simulink model "TCMSSystem"  (R2019b)
settings: configuration reference "ConfigSet_TCMSSystem_Reference" (kept outside this file)
model workspace (MAT data in the model file):
  Prm_TCMSSystem : Simulink.Parameter (value not decoded)
  SampleTime = 0.05
symbols that are objects in the model workspace (value not decoded): Prm_TCMSSystem
undefined symbols (not defined in the file): ADDIntervention, AK1Status, AK2Status, AKContactorStatus, AllDoorsClosed, AllLeftDoorsClosed, AllRightDoorsClosed, APS1Fault, APS1Isolated, APS1OutputVoltage, APS1Status, APS2Fault, APS2Isolated, APS2OutputVoltage, APS2Status, APSKAKContactor, ASCOEnd1, ASCOEnd2, ATBMode, ATCBypassMode, ATCStatusNotOK, ATOMode, ATPLowSpeedCutoutStatus, ATPMode, AuxCompressor, BatteryCurrent, BatteryIsolationContactor, BatteryTemperature, BatteryVoltage, BCG1Fault, BCG1Isolated, BCG1IsolationFailed, BCG1OutputCurrent, BCG1Status, BCG2Fault, BCG2Isolated, BCG2OutputCurrent, BCG2Status, BCGOutputVoltage, BECU1AxleLockedWheelSet1, BECU2AxleLockedWheelSet2, BECUFaulty, BECUMajorFault, BECUMinorFault, BECUStatus, BIC1Inside, BIC1Outside, BIC2Inside, BIC2Outside, Bogie, Bogie1WSPStatus, Bogie2WSPStatus, BogieFaulty, BogieIsolationStatus, BogieSupportedMass, BrakeCylinderPressureGauge, BrakeLoopCBTripped, BrakeLoopOpenTL, BrakeTrainLineStatus, BrakingDemand ... (+215)
libraries: TimersLib x257, simulink x137, LatchesLib x42, VectorOperationsLib x15, TestBenchLib x12, MathOperationsLib x2, FiltersLib x1
(part 10 of 16)

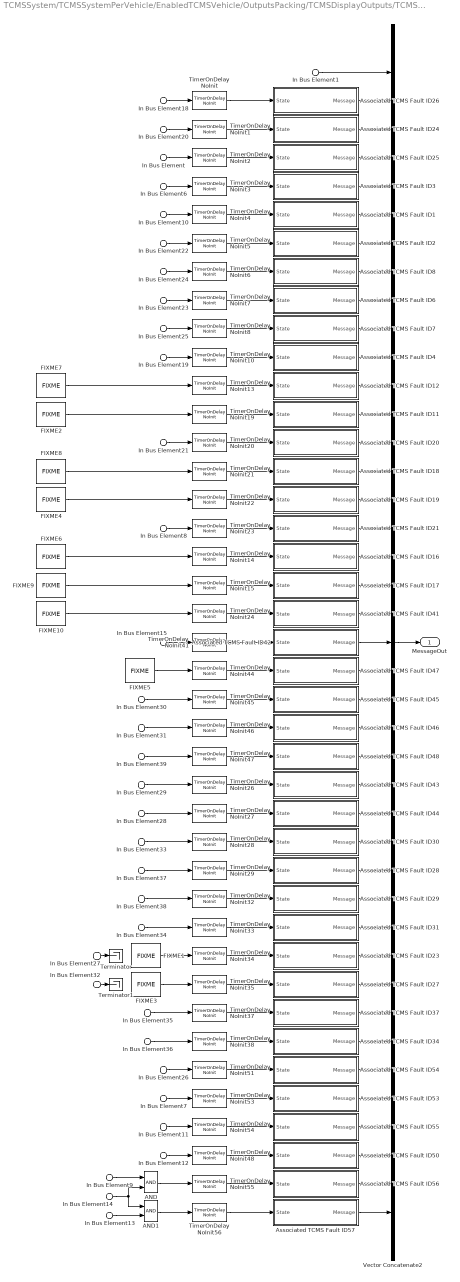
== system TCMSSystem/TCMSSystemPerVehicle/EnabledTCMSVehicle/OutputsPacking/TCMSDisplayOutputs/TCMSMessageEvents/New46EventsMessage ==
  In Bus Element1 : Inport  PortName=MessageIn
  In Bus Element15 : Inport  Port=2  PortName=BusIn  Element=PantographSystem.PantographIsolated
  In Bus Element : Inport  Port=2  PortName=BusIn  Element=ElectricalSystem.BrakeLoopCBTripped
  In Bus Element12 : Inport  Port=2  PortName=BusIn  Element=ElectricalSystem.VCBIsolated
  In Bus Element19 : Inport  Port=2  PortName=BusIn  Element=ElectricalSystem.APS2Isolated
  In Bus Element14 : Inport  Port=2  PortName=BusIn  Element=ElectricalSystem.CabActive
  In Bus Element6 : Inport  Port=2  PortName=BusIn  Element=PneumaticsSystem.Bogie1ParkingBrakeIsolated
  In Bus Element10 : Inport  Port=2  PortName=BusIn  Element=PneumaticsSystem.Bogie2ParkingBrakeIsolated
  In Bus Element8 : Inport  Port=3  PortName=ElectricalControl  Element=BLCOSwitchStatus
  In Bus Element9 : Inport  Port=3  PortName=ElectricalControl  Element=TooManyBogiesIsolated
  In Bus Element13 : Inport  Port=3  PortName=ElectricalControl  Element=TooManyEPICCutout
  In Bus Element26 : Inport  Port=3  PortName=ElectricalControl  Element=WFLIsolated
  In Bus Element27 : Inport  Port=3  PortName=ElectricalControl  Element=HVAC1FireDetectorDisableVDUReq
  In Bus Element28 : Inport  Port=3  PortName=ElectricalControl  Element=EDBHeatAlarmDisableVDUReq
  In Bus Element29 : Inport  Port=3  PortName=ElectricalControl  Element=CABSmokeDetectorDisableVDUReq
  In Bus Element30 : Inport  Port=3  PortName=ElectricalControl  Element=SHDEndCubicleRearRight1DisableVDUReq
  In Bus Element31 : Inport  Port=3  PortName=ElectricalControl  Element=SHDEndCubicleRearRight2DisableVDUReq
  In Bus Element32 : Inport  Port=3  PortName=ElectricalControl  Element=SHDEndCubicleRearLeft1DisableVDUReq
  In Bus Element33 : Inport  Port=3  PortName=ElectricalControl  Element=SHDEndCubicleRearLeft2DisableVDUReq
  In Bus Element34 : Inport  Port=3  PortName=ElectricalControl  Element=LHDDriverDeskDisableVDUReq
  In Bus Element35 : Inport  Port=3  PortName=ElectricalControl  Element=LHDCIDisableVDUReq
  In Bus Element36 : Inport  Port=3  PortName=ElectricalControl  Element=LHDLTJBDisableVDUReq
  In Bus Element37 : Inport  Port=3  PortName=ElectricalControl  Element=SaloonR1FireDetectorDisableVDUReq
  In Bus Element38 : Inport  Port=3  PortName=ElectricalControl  Element=SaloonR2FireDetectorDisableVDUReq
  In Bus Element39 : Inport  Port=3  PortName=ElectricalControl  Element=AuxiliaryDeskFireDetectorDisableVDUReq
  In Bus Element7 : Inport  Port=3  PortName=ElectricalControl  Element=RemoteMagnetValve1
  In Bus Element11 : Inport  Port=3  PortName=ElectricalControl  Element=RemoteMagnetValve2
  In Bus Element18 : Inport  Port=4  PortName=PneumaticsControl  Element=ASCOEnd1
  In Bus Element20 : Inport  Port=4  PortName=PneumaticsControl  Element=ASCOEnd2
  In Bus Element21 : Inport  Port=4  PortName=PneumaticsControl  Element=HornManuallyIsolated
  In Bus Element22 : Inport  Port=4  PortName=PneumaticsControl  Element=BIC1Inside
  In Bus Element23 : Inport  Port=4  PortName=PneumaticsControl  Element=BIC1Outside
  In Bus Element24 : Inport  Port=4  PortName=PneumaticsControl  Element=BIC2Inside
  In Bus Element25 : Inport  Port=4  PortName=PneumaticsControl  Element=BIC2Outside
  AND : Logic  AllPortsSameDT=off  OutDataTypeStr=boolean
  AND1 : Logic  AllPortsSameDT=off  OutDataTypeStr=boolean
  Associated TCMS Fault ID1 : Subsystem  mask{MessageID=91031}
      mask Display:
      | port_label('output', 1, ['ID = ' num2str(MessageID)])
      | port_label('input', 1, 'Status')
  Associated TCMS Fault ID11 : Subsystem  mask{MessageID=3006}
      mask Display:
      | port_label('output', 1, ['ID = ' num2str(MessageID)])
      | port_label('input', 1, 'Status')
  Associated TCMS Fault ID12 : Subsystem  mask{MessageID=241003}
      mask Display:
      | port_label('output', 1, ['ID = ' num2str(MessageID)])
      | port_label('input', 1, 'Status')
  Associated TCMS Fault ID16 : Subsystem  mask{MessageID=91044}
      mask Display:
      | port_label('output', 1, ['ID = ' num2str(MessageID)])
      | port_label('input', 1, 'Status')
  Associated TCMS Fault ID17 : Subsystem  mask{MessageID=12103}
      mask Display:
      | port_label('output', 1, ['ID = ' num2str(MessageID)])
      | port_label('input', 1, 'Status')
  Associated TCMS Fault ID18 : Subsystem  mask{MessageID=1010}
      mask Display:
      | port_label('output', 1, ['ID = ' num2str(MessageID)])
      | port_label('input', 1, 'Status')
  Associated TCMS Fault ID19 : Subsystem  mask{MessageID=1008}
      mask Display:
      | port_label('output', 1, ['ID = ' num2str(MessageID)])
      | port_label('input', 1, 'Status')
  Associated TCMS Fault ID2 : Subsystem  mask{MessageID=91026}
      mask Display:
      | port_label('output', 1, ['ID = ' num2str(MessageID)])
      | port_label('input', 1, 'Status')
  Associated TCMS Fault ID20 : Subsystem  mask{MessageID=1009}
      mask Display:
      | port_label('output', 1, ['ID = ' num2str(MessageID)])
      | port_label('input', 1, 'Status')
  Associated TCMS Fault ID21 : Subsystem  mask{MessageID=91022}
      mask Display:
      | port_label('output', 1, ['ID = ' num2str(MessageID)])
      | port_label('input', 1, 'Status')
  Associated TCMS Fault ID23 : Subsystem  mask{MessageID=151078}
      mask Display:
      | port_label('output', 1, ['ID = ' num2str(MessageID)])
      | port_label('input', 1, 'Status')
  Associated TCMS Fault ID24 : Subsystem  mask{MessageID=91033}
      mask Display:
      | port_label('output', 1, ['ID = ' num2str(MessageID)])
      | port_label('input', 1, 'Status')
  Associated TCMS Fault ID25 : Subsystem  mask{MessageID=93055}
      mask Display:
      | port_label('output', 1, ['ID = ' num2str(MessageID)])
      | port_label('input', 1, 'Status')
  Associated TCMS Fault ID26 : Subsystem  mask{MessageID=91032}
      mask Display:
      | port_label('output', 1, ['ID = ' num2str(MessageID)])
      | port_label('input', 1, 'Status')
  Associated TCMS Fault ID27 : Subsystem  mask{MessageID=151079}
      mask Display:
      | port_label('output', 1, ['ID = ' num2str(MessageID)])
      | port_label('input', 1, 'Status')
  Associated TCMS Fault ID28 : Subsystem  mask{MessageID=151067}
      mask Display:
      | port_label('output', 1, ['ID = ' num2str(MessageID)])
      | port_label('input', 1, 'Status')
  Associated TCMS Fault ID29 : Subsystem  mask{MessageID=151068}
      mask Display:
      | port_label('output', 1, ['ID = ' num2str(MessageID)])
      | port_label('input', 1, 'Status')
  Associated TCMS Fault ID3 : Subsystem  mask{MessageID=91030}
      mask Display:
      | port_label('output', 1, ['ID = ' num2str(MessageID)])
      | port_label('input', 1, 'Status')
  Associated TCMS Fault ID30 : Subsystem  mask{MessageID=151066}
      mask Display:
      | port_label('output', 1, ['ID = ' num2str(MessageID)])
      | port_label('input', 1, 'Status')
  Associated TCMS Fault ID31 : Subsystem  mask{MessageID=151077}
      mask Display:
      | port_label('output', 1, ['ID = ' num2str(MessageID)])
      | port_label('input', 1, 'Status')
  Associated TCMS Fault ID34 : Subsystem  mask{MessageID=151090}
      mask Display:
      | port_label('output', 1, ['ID = ' num2str(MessageID)])
      | port_label('input', 1, 'Status')
  Associated TCMS Fault ID37 : Subsystem  mask{MessageID=151089}
      mask Display:
      | port_label('output', 1, ['ID = ' num2str(MessageID)])
      | port_label('input', 1, 'Status')
  Associated TCMS Fault ID4 : Subsystem  mask{MessageID=232005}
      mask Display:
      | port_label('output', 1, ['ID = ' num2str(MessageID)])
      | port_label('input', 1, 'Status')
  Associated TCMS Fault ID41 : Subsystem  mask{MessageID=12104}
      mask Display:
      | port_label('output', 1, ['ID = ' num2str(MessageID)])
      | port_label('input', 1, 'Status')
  Associated TCMS Fault ID42 : Subsystem  mask{MessageID=12007}
      mask Display:
      | port_label('output', 1, ['ID = ' num2str(MessageID)])
      | port_label('input', 1, 'Status')
  Associated TCMS Fault ID43 : Subsystem  mask{MessageID=151064}
      mask Display:
      | port_label('output', 1, ['ID = ' num2str(MessageID)])
      | port_label('input', 1, 'Status')
  Associated TCMS Fault ID44 : Subsystem  mask{MessageID=151065}
      mask Display:
      | port_label('output', 1, ['ID = ' num2str(MessageID)])
      | port_label('input', 1, 'Status')
  Associated TCMS Fault ID45 : Subsystem  mask{MessageID=151061}
      mask Display:
      | port_label('output', 1, ['ID = ' num2str(MessageID)])
      | port_label('input', 1, 'Status')
  Associated TCMS Fault ID46 : Subsystem  mask{MessageID=151062}
      mask Display:
      | port_label('output', 1, ['ID = ' num2str(MessageID)])
      | port_label('input', 1, 'Status')
  Associated TCMS Fault ID47 : Subsystem  mask{MessageID=30035}
      mask Display:
      | port_label('output', 1, ['ID = ' num2str(MessageID)])
      | port_label('input', 1, 'Status')
  Associated TCMS Fault ID48 : Subsystem  mask{MessageID=151063}
      mask Display:
      | port_label('output', 1, ['ID = ' num2str(MessageID)])
      | port_label('input', 1, 'Status')
  Associated TCMS Fault ID50 : Subsystem  mask{MessageID=12014}
      mask Display:
      | port_label('output', 1, ['ID = ' num2str(MessageID)])
      | port_label('input', 1, 'Status')
  Associated TCMS Fault ID53 : Subsystem  mask{MessageID=91036}
      mask Display:
      | port_label('output', 1, ['ID = ' num2str(MessageID)])
      | port_label('input', 1, 'Status')
  Associated TCMS Fault ID54 : Subsystem  mask{MessageID=261006}
      mask Display:
      | port_label('output', 1, ['ID = ' num2str(MessageID)])
      | port_label('input', 1, 'Status')
  Associated TCMS Fault ID55 : Subsystem  mask{MessageID=91037}
      mask Display:
      | port_label('output', 1, ['ID = ' num2str(MessageID)])
      | port_label('input', 1, 'Status')
  Associated TCMS Fault ID56 : Subsystem  mask{MessageID=888888}
      mask Display:
      | port_label('output', 1, ['ID = ' num2str(MessageID)])
      | port_label('input', 1, 'Status')
  Associated TCMS Fault ID57 : Subsystem  mask{MessageID=999999}
      mask Display:
      | port_label('output', 1, ['ID = ' num2str(MessageID)])
      | port_label('input', 1, 'Status')
  Associated TCMS Fault ID6 : Subsystem  mask{MessageID=91028}
      mask Display:
      | port_label('output', 1, ['ID = ' num2str(MessageID)])
      | port_label('input', 1, 'Status')
  Associated TCMS Fault ID7 : Subsystem  mask{MessageID=91029}
      mask Display:
      | port_label('output', 1, ['ID = ' num2str(MessageID)])
      | port_label('input', 1, 'Status')
  Associated TCMS Fault ID8 : Subsystem  mask{MessageID=91027}
      mask Display:
      | port_label('output', 1, ['ID = ' num2str(MessageID)])
      | port_label('input', 1, 'Status')
  FIXME{1..10} (10 alike) : TestBenchLib/FIXME
      settings: SourceProductName=Sydac Utilities
  Terminator : Terminator
  Terminator1 : Terminator
  TimerOnDelay NoInit{,1..8,10,13..15,19..24,26..29,32..35,37..38,41,44..48,51,53..56} (40 alike) : TimersLib/TimerOnDelay NoInit  UpperSaturationLimit=0.5  OutputTime=off  SampleTime=-1
      settings: SourceProductName=Sydac Utilities
  Vector Concatenate2 : Concatenate  NumInputs=41
  MessageOut : Outport
  wires:
  TimerOnDelay NoInit2/1 -> Associated TCMS Fault ID25/1(State)
  TimerOnDelay NoInit1/1 -> Associated TCMS Fault ID24/1(State)
  TimerOnDelay NoInit/1 -> Associated TCMS Fault ID26/1(State)
  In Bus Element1/1 -> Vector Concatenate2/1
  Associated TCMS Fault ID25/1(Message) -> Vector Concatenate2/4
  Associated TCMS Fault ID26/1(Message) -> Vector Concatenate2/2
  In Bus Element/1 -> TimerOnDelay NoInit2/1
  Vector Concatenate2/1 -> MessageOut/1
  Associated TCMS Fault ID24/1(Message) -> Vector Concatenate2/3
  Associated TCMS Fault ID1/1(Message) -> Vector Concatenate2/6
  Associated TCMS Fault ID3/1(Message) -> Vector Concatenate2/5
  Associated TCMS Fault ID2/1(Message) -> Vector Concatenate2/7
  TimerOnDelay NoInit3/1 -> Associated TCMS Fault ID3/1(State)
  TimerOnDelay NoInit4/1 -> Associated TCMS Fault ID1/1(State)
  TimerOnDelay NoInit5/1 -> Associated TCMS Fault ID2/1(State)
  TimerOnDelay NoInit10/1 -> Associated TCMS Fault ID4/1(State)
  In Bus Element19/1 -> TimerOnDelay NoInit10/1
  Associated TCMS Fault ID6/1(Message) -> Vector Concatenate2/9
  Associated TCMS Fault ID8/1(Message) -> Vector Concatenate2/8
  Associated TCMS Fault ID7/1(Message) -> Vector Concatenate2/10
  TimerOnDelay NoInit6/1 -> Associated TCMS Fault ID8/1(State)
  TimerOnDelay NoInit7/1 -> Associated TCMS Fault ID6/1(State)
  TimerOnDelay NoInit8/1 -> Associated TCMS Fault ID7/1(State)
  TimerOnDelay NoInit22/1 -> Associated TCMS Fault ID19/1(State)
  TimerOnDelay NoInit21/1 -> Associated TCMS Fault ID18/1(State)
  TimerOnDelay NoInit20/1 -> Associated TCMS Fault ID20/1(State)
  FIXME2/1 -> TimerOnDelay NoInit19/1
  FIXME8/1 -> TimerOnDelay NoInit21/1
  FIXME6/1 -> TimerOnDelay NoInit14/1
  FIXME9/1 -> TimerOnDelay NoInit15/1
  TimerOnDelay NoInit23/1 -> Associated TCMS Fault ID21/1(State)
  TimerOnDelay NoInit14/1 -> Associated TCMS Fault ID16/1(State)
  TimerOnDelay NoInit15/1 -> Associated TCMS Fault ID17/1(State)
  TimerOnDelay NoInit19/1 -> Associated TCMS Fault ID11/1(State)
  FIXME7/1 -> TimerOnDelay NoInit13/1
  TimerOnDelay NoInit13/1 -> Associated TCMS Fault ID12/1(State)
  TimerOnDelay NoInit32/1 -> Associated TCMS Fault ID29/1(State)
  TimerOnDelay NoInit29/1 -> Associated TCMS Fault ID28/1(State)
  TimerOnDelay NoInit28/1 -> Associated TCMS Fault ID30/1(State)
  TimerOnDelay NoInit33/1 -> Associated TCMS Fault ID31/1(State)
  TimerOnDelay NoInit34/1 -> Associated TCMS Fault ID23/1(State)
  TimerOnDelay NoInit35/1 -> Associated TCMS Fault ID27/1(State)
  FIXME5/1 -> TimerOnDelay NoInit44/1
  TimerOnDelay NoInit37/1 -> Associated TCMS Fault ID37/1(State)
  TimerOnDelay NoInit38/1 -> Associated TCMS Fault ID34/1(State)
  TimerOnDelay NoInit46/1 -> Associated TCMS Fault ID46/1(State)
  TimerOnDelay NoInit45/1 -> Associated TCMS Fault ID45/1(State)
  TimerOnDelay NoInit44/1 -> Associated TCMS Fault ID47/1(State)
  TimerOnDelay NoInit47/1 -> Associated TCMS Fault ID48/1(State)
  TimerOnDelay NoInit26/1 -> Associated TCMS Fault ID43/1(State)
  TimerOnDelay NoInit27/1 -> Associated TCMS Fault ID44/1(State)
  TimerOnDelay NoInit41/1 -> Associated TCMS Fault ID42/1(State)
  TimerOnDelay NoInit24/1 -> Associated TCMS Fault ID41/1(State)
  TimerOnDelay NoInit53/1 -> Associated TCMS Fault ID53/1(State)
  TimerOnDelay NoInit51/1 -> Associated TCMS Fault ID54/1(State)
  TimerOnDelay NoInit54/1 -> Associated TCMS Fault ID55/1(State)
  TimerOnDelay NoInit48/1 -> Associated TCMS Fault ID50/1(State)
  TimerOnDelay NoInit56/1 -> Associated TCMS Fault ID57/1(State)
  TimerOnDelay NoInit55/1 -> Associated TCMS Fault ID56/1(State)
  Associated TCMS Fault ID4/1(Message) -> Vector Concatenate2/11
  Associated TCMS Fault ID12/1(Message) -> Vector Concatenate2/12
  Associated TCMS Fault ID11/1(Message) -> Vector Concatenate2/13
  Associated TCMS Fault ID20/1(Message) -> Vector Concatenate2/14
  Associated TCMS Fault ID18/1(Message) -> Vector Concatenate2/15
  Associated TCMS Fault ID19/1(Message) -> Vector Concatenate2/16
  Associated TCMS Fault ID21/1(Message) -> Vector Concatenate2/17
  Associated TCMS Fault ID16/1(Message) -> Vector Concatenate2/18
  Associated TCMS Fault ID17/1(Message) -> Vector Concatenate2/19
  Associated TCMS Fault ID41/1(Message) -> Vector Concatenate2/20
  Associated TCMS Fault ID42/1(Message) -> Vector Concatenate2/21
  Associated TCMS Fault ID47/1(Message) -> Vector Concatenate2/22
  Associated TCMS Fault ID45/1(Message) -> Vector Concatenate2/23
  Associated TCMS Fault ID46/1(Message) -> Vector Concatenate2/24
  Associated TCMS Fault ID48/1(Message) -> Vector Concatenate2/25
  Associated TCMS Fault ID43/1(Message) -> Vector Concatenate2/26
  Associated TCMS Fault ID44/1(Message) -> Vector Concatenate2/27
  Associated TCMS Fault ID30/1(Message) -> Vector Concatenate2/28
  Associated TCMS Fault ID28/1(Message) -> Vector Concatenate2/29
  Associated TCMS Fault ID29/1(Message) -> Vector Concatenate2/30
  Associated TCMS Fault ID31/1(Message) -> Vector Concatenate2/31
  Associated TCMS Fault ID23/1(Message) -> Vector Concatenate2/32
  Associated TCMS Fault ID27/1(Message) -> Vector Concatenate2/33
  Associated TCMS Fault ID37/1(Message) -> Vector Concatenate2/34
  Associated TCMS Fault ID34/1(Message) -> Vector Concatenate2/35
  Associated TCMS Fault ID54/1(Message) -> Vector Concatenate2/36
  Associated TCMS Fault ID53/1(Message) -> Vector Concatenate2/37
  Associated TCMS Fault ID55/1(Message) -> Vector Concatenate2/38
  Associated TCMS Fault ID50/1(Message) -> Vector Concatenate2/39
  Associated TCMS Fault ID56/1(Message) -> Vector Concatenate2/40
  Associated TCMS Fault ID57/1(Message) -> Vector Concatenate2/41
  In Bus Element6/1 -> TimerOnDelay NoInit3/1
  In Bus Element10/1 -> TimerOnDelay NoInit4/1
  In Bus Element15/1 -> TimerOnDelay NoInit41/1
  In Bus Element7/1 -> TimerOnDelay NoInit53/1
  In Bus Element11/1 -> TimerOnDelay NoInit54/1
  FIXME10/1 -> TimerOnDelay NoInit24/1
  In Bus Element12/1 -> TimerOnDelay NoInit48/1
  FIXME4/1 -> TimerOnDelay NoInit22/1
  In Bus Element8/1 -> TimerOnDelay NoInit23/1
  In Bus Element9/1 -> AND/1
  In Bus Element13/1 -> AND1/2
  In Bus Element14/1 -> AND1/1, AND/2
  AND/1 -> TimerOnDelay NoInit55/1
  AND1/1 -> TimerOnDelay NoInit56/1
  In Bus Element18/1 -> TimerOnDelay NoInit/1
  In Bus Element20/1 -> TimerOnDelay NoInit1/1
  In Bus Element21/1 -> TimerOnDelay NoInit20/1
  In Bus Element22/1 -> TimerOnDelay NoInit5/1
  In Bus Element23/1 -> TimerOnDelay NoInit7/1
  In Bus Element24/1 -> TimerOnDelay NoInit6/1
  In Bus Element25/1 -> TimerOnDelay NoInit8/1
  In Bus Element26/1 -> TimerOnDelay NoInit51/1
  In Bus Element30/1 -> TimerOnDelay NoInit45/1
  In Bus Element31/1 -> TimerOnDelay NoInit46/1
  In Bus Element39/1 -> TimerOnDelay NoInit47/1
  In Bus Element29/1 -> TimerOnDelay NoInit26/1
  In Bus Element28/1 -> TimerOnDelay NoInit27/1
  In Bus Element33/1 -> TimerOnDelay NoInit28/1
  In Bus Element37/1 -> TimerOnDelay NoInit29/1
  In Bus Element38/1 -> TimerOnDelay NoInit32/1
  In Bus Element34/1 -> TimerOnDelay NoInit33/1
  In Bus Element35/1 -> TimerOnDelay NoInit37/1
  In Bus Element36/1 -> TimerOnDelay NoInit38/1
  FIXME1/1 -> TimerOnDelay NoInit34/1
  FIXME3/1 -> TimerOnDelay NoInit35/1
  In Bus Element27/1 -> Terminator/1
  In Bus Element32/1 -> Terminator1/1

== system TCMSSystem/TCMSSystemPerVehicle/EnabledTCMSVehicle/OutputsPacking/TCMSDisplayOutputs/TCMSMessageEvents/PantographSystemFaults ==
  note: Pantograph Faults
  note: Pantograph ADD
  note: Pantograph ORD
  note: Pantograph Raise Failure
  In Bus Element1 : Inport  PortName=MessageIn
  In Bus Element24 : Inport  Port=2  PortName=BusIn  Element=PantographSystem.PantoADDFaultMessage
  In Bus Element25 : Inport  Port=2  PortName=BusIn  Element=PantographSystem.PantoORDFaultMessage
  In Bus Element26 : Inport  Port=2  PortName=BusIn  Element=PantographSystem.PantoRaiseFailureMessage
  Associated TCMS Fault ID24 : Subsystem  mask{MessageID=012002}
      mask Display:
      | port_label('output', 1, ['ID = ' num2str(MessageID)])
      | port_label('input', 1, 'Status')
  Associated TCMS Fault ID25 : Subsystem  mask{MessageID=012021}
      mask Display:
      | port_label('output', 1, ['ID = ' num2str(MessageID)])
      | port_label('input', 1, 'Status')
  Associated TCMS Fault ID26 : Subsystem  mask{MessageID=012001}
      mask Display:
      | port_label('output', 1, ['ID = ' num2str(MessageID)])
      | port_label('input', 1, 'Status')
  TimerOnDelay NoInit : TimersLib/TimerOnDelay NoInit  UpperSaturationLimit=0.5  OutputTime=off  SampleTime=-1
      settings: SourceProductName=Sydac Utilities
  TimerOnDelay NoInit1 : TimersLib/TimerOnDelay NoInit  UpperSaturationLimit=0.5  OutputTime=off  SampleTime=-1
      settings: SourceProductName=Sydac Utilities
  TimerOnDelay NoInit2 : TimersLib/TimerOnDelay NoInit  UpperSaturationLimit=0.5  OutputTime=off  SampleTime=-1
      settings: SourceProductName=Sydac Utilities
  Vector Concatenate2 : Concatenate  NumInputs=4
  MessageOut : Outport
  wires:
  Associated TCMS Fault ID24/1(Message) -> Vector Concatenate2/3
  Vector Concatenate2/1 -> MessageOut/1
  In Bus Element25/1 -> TimerOnDelay NoInit1/1
  In Bus Element26/1 -> TimerOnDelay NoInit2/1
  Associated TCMS Fault ID26/1(Message) -> Vector Concatenate2/2
  In Bus Element24/1 -> TimerOnDelay NoInit/1
  Associated TCMS Fault ID25/1(Message) -> Vector Concatenate2/4
  In Bus Element1/1 -> Vector Concatenate2/1
  TimerOnDelay NoInit/1 -> Associated TCMS Fault ID26/1(State)
  TimerOnDelay NoInit1/1 -> Associated TCMS Fault ID24/1(State)
  TimerOnDelay NoInit2/1 -> Associated TCMS Fault ID25/1(State)

== system TCMSSystem/TCMSSystemPerVehicle/EnabledTCMSVehicle/OutputsPacking/TCMSDisplayOutputs/TCMSMessageEvents/TCMSSystemFaults ==
  note: MCandTrainLineIncongruence
  note: TCMS Faults
  note: MCB TCMS Group Open
  note: RIO Mastership error
  note: ER Fault
  note: Communication RIO1 and RIO2 fault
  note: CCU Communication Error
  In Bus Element : Inport  PortName=MessageIn
  In Bus Element7 : Inport  Port=2  PortName=BusIn  Element=TCMSSystem.RemoteHornIsolated
  In Bus Element3 : Inport  Port=2  PortName=BusIn  Element=TCMSSystem.CCUFault
  In Bus Element5 : Inport  Port=2  PortName=BusIn  Element=TCMSSystem.RIO1Fault
  In Bus Element8 : Inport  Port=2  PortName=BusIn  Element=TCMSSystem.RIO1RIO2Fault
  In Bus Element9 : Inport  Port=2  PortName=BusIn  Element=TCMSSystem.ERFault
  In Bus Element20 : Inport  Port=3  PortName=TCMSFaults  Element=MasterControllerandTrainLineIncongruence
  In Bus Element4 : Inport  Port=4  PortName=ElectricalControl  Element=MCBTCMSGroup
  In Bus Element1 : Inport  Port=5  PortName=TractionControl  Element=TractionCutModeSelectorInATPATOUTO
  Associated TCMS Fault ID1 : Subsystem  mask{MessageID=041001}
      mask Display:
      | port_label('output', 1, ['ID = ' num2str(MessageID)])
      | port_label('input', 1, 'Status')
  Associated TCMS Fault ID100 : Subsystem  mask{MessageID=041003}
      mask Display:
      | port_label('output', 1, ['ID = ' num2str(MessageID)])
      | port_label('input', 1, 'Status')
  Associated TCMS Fault ID101 : Subsystem  mask{MessageID=041140}
      mask Display:
      | port_label('output', 1, ['ID = ' num2str(MessageID)])
      | port_label('input', 1, 'Status')
  Associated TCMS Fault ID21 : Subsystem  mask{MessageID=031104}
      mask Display:
      | port_label('output', 1, ['ID = ' num2str(MessageID)])
      | port_label('input', 1, 'Status')
  Associated TCMS Fault ID97 : Subsystem  mask{MessageID=040004}
      mask Display:
      | port_label('output', 1, ['ID = ' num2str(MessageID)])
      | port_label('input', 1, 'Status')
  Associated TCMS Fault ID98 : Subsystem  mask{MessageID=041002}
      mask Display:
      | port_label('output', 1, ['ID = ' num2str(MessageID)])
      | port_label('input', 1, 'Status')
  Associated TCMS Fault ID99 : Subsystem  mask{MessageID=120002}
      mask Display:
      | port_label('output', 1, ['ID = ' num2str(MessageID)])
      | port_label('input', 1, 'Status')
  Terminator : Terminator
  TimerOnDelay NoInit{1..7} (7 alike) : TimersLib/TimerOnDelay NoInit  UpperSaturationLimit=0.5  OutputTime=off  SampleTime=-1
      settings: SourceProductName=Sydac Utilities
  Vector Concatenate4 : Concatenate  NumInputs=8
  MessageOut : Outport
  wires:
  Associated TCMS Fault ID100/1(Message) -> Vector Concatenate4/6
  Associated TCMS Fault ID21/1(Message) -> Vector Concatenate4/2
  Associated TCMS Fault ID97/1(Message) -> Vector Concatenate4/4
  Associated TCMS Fault ID101/1(Message) -> Vector Concatenate4/7
  In Bus Element20/1 -> TimerOnDelay NoInit2/1
  Associated TCMS Fault ID98/1(Message) -> Vector Concatenate4/5
  Associated TCMS Fault ID99/1(Message) -> Vector Concatenate4/3
  Vector Concatenate4/1 -> MessageOut/1
  In Bus Element/1 -> Vector Concatenate4/1
  In Bus Element1/1 -> TimerOnDelay NoInit1/1
  In Bus Element3/1 -> TimerOnDelay NoInit3/1
  In Bus Element8/1 -> TimerOnDelay NoInit4/1
  In Bus Element4/1 -> TimerOnDelay NoInit5/1
  In Bus Element9/1 -> TimerOnDelay NoInit6/1
  In Bus Element7/1 -> Terminator/1
  In Bus Element5/1 -> TimerOnDelay NoInit7/1
  Associated TCMS Fault ID1/1(Message) -> Vector Concatenate4/8
  TimerOnDelay NoInit2/1 -> Associated TCMS Fault ID21/1(State)
  TimerOnDelay NoInit1/1 -> Associated TCMS Fault ID99/1(State)
  TimerOnDelay NoInit3/1 -> Associated TCMS Fault ID97/1(State)
  TimerOnDelay NoInit4/1 -> Associated TCMS Fault ID98/1(State)
  TimerOnDelay NoInit5/1 -> Associated TCMS Fault ID100/1(State)
  TimerOnDelay NoInit6/1 -> Associated TCMS Fault ID101/1(State)
  TimerOnDelay NoInit7/1 -> Associated TCMS Fault ID1/1(State)

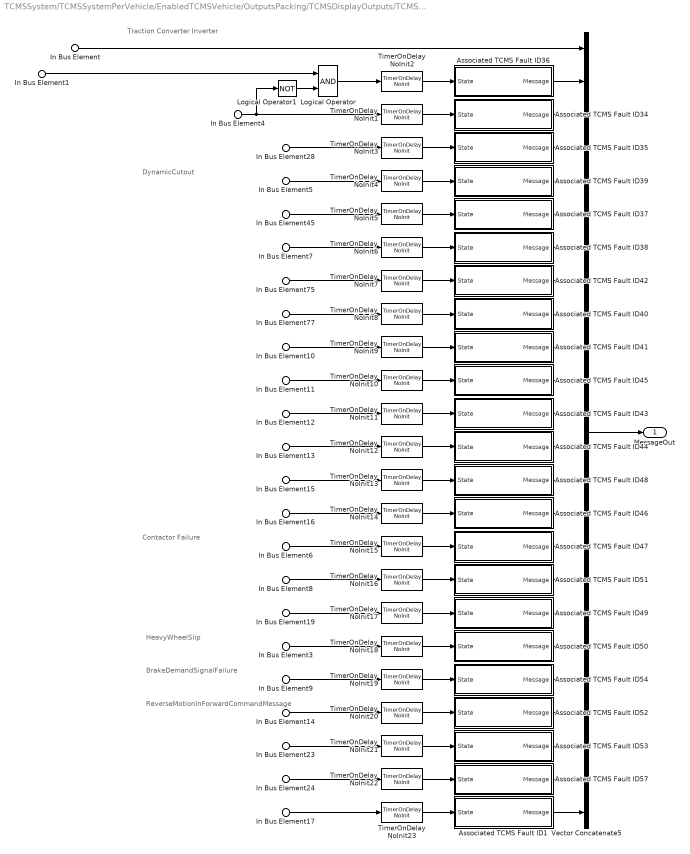
== system TCMSSystem/TCMSSystemPerVehicle/EnabledTCMSVehicle/OutputsPacking/TCMSDisplayOutputs/TCMSMessageEvents/TractionSystemFaults ==
  note: Traction Converter Inverter
  note: ReverseMotionInForwardCommandMessage
  note: HeavyWheelSlip
  note: DynamicCutout
  note: Contactor Failure
  note: BrakeDemandSignalFailure
  In Bus Element : Inport  PortName=MessageIn
  In Bus Element3 : Inport  Port=2  PortName=BusIn  Element=TractionBraking.HeavyWheelSlipDetected
  In Bus Element5 : Inport  Port=2  PortName=BusIn  Element=TractionBraking.DynamicBrakeCutoutDueToSlide
  In Bus Element14 : Inport  Port=2  PortName=BusIn  Element=TractionBraking.RollbackDetected
  In Bus Element17 : Inport  Port=2  PortName=BusIn  Element=TractionBraking.HTERequired
  In Bus Element9 : Inport  Port=2  PortName=BusIn  Element=PneumaticsSystem.BrakeDemandSignalFailure
  In Bus Element1 : Inport  Port=3  PortName=VehicleLevelFaults  Element=CIFailure
  In Bus Element7 : Inport  Port=3  PortName=VehicleLevelFaults  Element=LineConverterOverCurrentLevel2
  In Bus Element10 : Inport  Port=3  PortName=VehicleLevelFaults  Element=LineConverterIGBTFailure
  In Bus Element11 : Inport  Port=3  PortName=VehicleLevelFaults  Element=DC110VLowVoltage
  In Bus Element12 : Inport  Port=3  PortName=VehicleLevelFaults  Element=CIMicroprocessorAbnormal
  In Bus Element13 : Inport  Port=3  PortName=VehicleLevelFaults  Element=CILocalCommunicationFailure
  In Bus Element15 : Inport  Port=3  PortName=VehicleLevelFaults  Element=OverTemperatureOfInverterPowerUnit
  In Bus Element16 : Inport  Port=3  PortName=VehicleLevelFaults  Element=OverTemperatureOfConverterPowerUnit
  In Bus Element19 : Inport  Port=3  PortName=VehicleLevelFaults  Element=MainCircuitEarthFaultLevel2
  In Bus Element23 : Inport  Port=3  PortName=VehicleLevelFaults  Element=CIGateSignalAbnormal
  In Bus Element24 : Inport  Port=3  PortName=VehicleLevelFaults  Element=CITCMSCommunicationFailure
  In Bus Element28 : Inport  Port=4  PortName=ElectricalControl  Element=OHLHighVoltageLevel3
  In Bus Element45 : Inport  Port=4  PortName=ElectricalControl  Element=OHLLowVoltageLevel2
  In Bus Element75 : Inport  Port=4  PortName=ElectricalControl  Element=DCLinkOverVoltageLevel1
  In Bus Element77 : Inport  Port=4  PortName=ElectricalControl  Element=DCLinkLowVoltageLevel1
  In Bus Element6 : Inport  Port=4  PortName=ElectricalControl  Element=AKOpenFailure
  In Bus Element8 : Inport  Port=4  PortName=ElectricalControl  Element=KOpenFailure
  In Bus Element4 : Inport  Port=5  PortName=TractionControl  Element=CIIsolated
  Associated TCMS Fault ID1 : Subsystem  mask{MessageID=241005}
      mask Display:
      | port_label('output', 1, ['ID = ' num2str(MessageID)])
      | port_label('input', 1, 'Status')
  Associated TCMS Fault ID34 : Subsystem  mask{MessageID=241003}
      mask Display:
      | port_label('output', 1, ['ID = ' num2str(MessageID)])
      | port_label('input', 1, 'Status')
  Associated TCMS Fault ID35 : Subsystem  mask{MessageID=241110}
      mask Display:
      | port_label('output', 1, ['ID = ' num2str(MessageID)])
      | port_label('input', 1, 'Status')
  Associated TCMS Fault ID36 : Subsystem  mask{MessageID=241001}
      mask Display:
      | port_label('output', 1, ['ID = ' num2str(MessageID)])
      | port_label('input', 1, 'Status')
  Associated TCMS Fault ID37 : Subsystem  mask{MessageID=241120}
      mask Display:
      | port_label('output', 1, ['ID = ' num2str(MessageID)])
      | port_label('input', 1, 'Status')
  Associated TCMS Fault ID38 : Subsystem  mask{MessageID=241123}
      mask Display:
      | port_label('output', 1, ['ID = ' num2str(MessageID)])
      | port_label('input', 1, 'Status')
  Associated TCMS Fault ID39 : Subsystem  mask{MessageID=241116}
      mask Display:
      | port_label('output', 1, ['ID = ' num2str(MessageID)])
      | port_label('input', 1, 'Status')
  Associated TCMS Fault ID40 : Subsystem  mask{MessageID=241126}
      mask Display:
      | port_label('output', 1, ['ID = ' num2str(MessageID)])
      | port_label('input', 1, 'Status')
  Associated TCMS Fault ID41 : Subsystem  mask{MessageID=241130}
      mask Display:
      | port_label('output', 1, ['ID = ' num2str(MessageID)])
      | port_label('input', 1, 'Status')
  Associated TCMS Fault ID42 : Subsystem  mask{MessageID=241124}
      mask Display:
      | port_label('output', 1, ['ID = ' num2str(MessageID)])
      | port_label('input', 1, 'Status')
  Associated TCMS Fault ID43 : Subsystem  mask{MessageID=241139}
      mask Display:
      | port_label('output', 1, ['ID = ' num2str(MessageID)])
      | port_label('input', 1, 'Status')
  Associated TCMS Fault ID44 : Subsystem  mask{MessageID=241141}
      mask Display:
      | port_label('output', 1, ['ID = ' num2str(MessageID)])
      | port_label('input', 1, 'Status')
  Associated TCMS Fault ID45 : Subsystem  mask{MessageID=241131}
      mask Display:
      | port_label('output', 1, ['ID = ' num2str(MessageID)])
      | port_label('input', 1, 'Status')
  Associated TCMS Fault ID46 : Subsystem  mask{MessageID=241145}
      mask Display:
      | port_label('output', 1, ['ID = ' num2str(MessageID)])
      | port_label('input', 1, 'Status')
  Associated TCMS Fault ID47 : Subsystem  mask{MessageID=241149}
      mask Display:
      | port_label('output', 1, ['ID = ' num2str(MessageID)])
      | port_label('input', 1, 'Status')
  Associated TCMS Fault ID48 : Subsystem  mask{MessageID=241143}
      mask Display:
      | port_label('output', 1, ['ID = ' num2str(MessageID)])
      | port_label('input', 1, 'Status')
  Associated TCMS Fault ID49 : Subsystem  mask{MessageID=241154}
      mask Display:
      | port_label('output', 1, ['ID = ' num2str(MessageID)])
      | port_label('input', 1, 'Status')
  Associated TCMS Fault ID50 : Subsystem  mask{MessageID=241155}
      mask Display:
      | port_label('output', 1, ['ID = ' num2str(MessageID)])
      | port_label('input', 1, 'Status')
  Associated TCMS Fault ID51 : Subsystem  mask{MessageID=241151}
      mask Display:
      | port_label('output', 1, ['ID = ' num2str(MessageID)])
      | port_label('input', 1, 'Status')
  Associated TCMS Fault ID52 : Subsystem  mask{MessageID=241157}
      mask Display:
      | port_label('output', 1, ['ID = ' num2str(MessageID)])
      | port_label('input', 1, 'Status')
  Associated TCMS Fault ID53 : Subsystem  mask{MessageID=241159}
      mask Display:
      | port_label('output', 1, ['ID = ' num2str(MessageID)])
      | port_label('input', 1, 'Status')
  Associated TCMS Fault ID54 : Subsystem  mask{MessageID=241156}
      mask Display:
      | port_label('output', 1, ['ID = ' num2str(MessageID)])
      | port_label('input', 1, 'Status')
  Associated TCMS Fault ID57 : Subsystem  mask{MessageID=241163}
      mask Display:
      | port_label('output', 1, ['ID = ' num2str(MessageID)])
      | port_label('input', 1, 'Status')
  Logical Operator : Logic  AllPortsSameDT=off  OutDataTypeStr=boolean
  Logical Operator1 : Logic  Operator=NOT  AllPortsSameDT=off  OutDataTypeStr=boolean
  TimerOnDelay NoInit{1..23} (23 alike) : TimersLib/TimerOnDelay NoInit  UpperSaturationLimit=0.5  OutputTime=off  SampleTime=-1
      settings: SourceProductName=Sydac Utilities
  Vector Concatenate5 : Concatenate  NumInputs=24
  MessageOut : Outport
  wires:
  Associated TCMS Fault ID46/1(Message) -> Vector Concatenate5/15
  Associated TCMS Fault ID51/1(Message) -> Vector Concatenate5/17
  Associated TCMS Fault ID35/1(Message) -> Vector Concatenate5/4
  Associated TCMS Fault ID47/1(Message) -> Vector Concatenate5/16
  Associated TCMS Fault ID42/1(Message) -> Vector Concatenate5/8
  Associated TCMS Fault ID38/1(Message) -> Vector Concatenate5/7
  Associated TCMS Fault ID34/1(Message) -> Vector Concatenate5/3
  Associated TCMS Fault ID44/1(Message) -> Vector Concatenate5/13
  Associated TCMS Fault ID45/1(Message) -> Vector Concatenate5/11
  Associated TCMS Fault ID53/1(Message) -> Vector Concatenate5/22
  Associated TCMS Fault ID43/1(Message) -> Vector Concatenate5/12
  Associated TCMS Fault ID41/1(Message) -> Vector Concatenate5/10
  Associated TCMS Fault ID57/1(Message) -> Vector Concatenate5/23
  Associated TCMS Fault ID52/1(Message) -> Vector Concatenate5/21
  Associated TCMS Fault ID50/1(Message) -> Vector Concatenate5/19
  Associated TCMS Fault ID49/1(Message) -> Vector Concatenate5/18
  Associated TCMS Fault ID48/1(Message) -> Vector Concatenate5/14
  Associated TCMS Fault ID54/1(Message) -> Vector Concatenate5/20
  Associated TCMS Fault ID37/1(Message) -> Vector Concatenate5/6
  Associated TCMS Fault ID40/1(Message) -> Vector Concatenate5/9
  Associated TCMS Fault ID36/1(Message) -> Vector Concatenate5/2
  Associated TCMS Fault ID39/1(Message) -> Vector Concatenate5/5
  Vector Concatenate5/1 -> MessageOut/1
  In Bus Element/1 -> Vector Concatenate5/1
  In Bus Element4/1 -> Logical Operator1/1, TimerOnDelay NoInit1/1
  In Bus Element1/1 -> Logical Operator/1
  In Bus Element28/1 -> TimerOnDelay NoInit3/1
  In Bus Element45/1 -> TimerOnDelay NoInit5/1
  In Bus Element7/1 -> TimerOnDelay NoInit6/1
  In Bus Element75/1 -> TimerOnDelay NoInit7/1
  In Bus Element77/1 -> TimerOnDelay NoInit8/1
  In Bus Element10/1 -> TimerOnDelay NoInit9/1
  In Bus Element11/1 -> TimerOnDelay NoInit10/1
  In Bus Element12/1 -> TimerOnDelay NoInit11/1
  In Bus Element13/1 -> TimerOnDelay NoInit12/1
  In Bus Element5/1 -> TimerOnDelay NoInit4/1
  In Bus Element15/1 -> TimerOnDelay NoInit13/1
  In Bus Element16/1 -> TimerOnDelay NoInit14/1
  In Bus Element6/1 -> TimerOnDelay NoInit15/1
  In Bus Element8/1 -> TimerOnDelay NoInit16/1
  In Bus Element19/1 -> TimerOnDelay NoInit17/1
  In Bus Element3/1 -> TimerOnDelay NoInit18/1
  In Bus Element9/1 -> TimerOnDelay NoInit19/1
  In Bus Element14/1 -> TimerOnDelay NoInit20/1
  In Bus Element23/1 -> TimerOnDelay NoInit21/1
  In Bus Element24/1 -> TimerOnDelay NoInit22/1
  Logical Operator/1 -> TimerOnDelay NoInit2/1
  Logical Operator1/1 -> Logical Operator/2
  Associated TCMS Fault ID1/1(Message) -> Vector Concatenate5/24
  In Bus Element17/1 -> TimerOnDelay NoInit23/1
  TimerOnDelay NoInit2/1 -> Associated TCMS Fault ID36/1(State)
  TimerOnDelay NoInit1/1 -> Associated TCMS Fault ID34/1(State)
  TimerOnDelay NoInit3/1 -> Associated TCMS Fault ID35/1(State)
  TimerOnDelay NoInit4/1 -> Associated TCMS Fault ID39/1(State)
  TimerOnDelay NoInit5/1 -> Associated TCMS Fault ID37/1(State)
  TimerOnDelay NoInit6/1 -> Associated TCMS Fault ID38/1(State)
  TimerOnDelay NoInit7/1 -> Associated TCMS Fault ID42/1(State)
  TimerOnDelay NoInit8/1 -> Associated TCMS Fault ID40/1(State)
  TimerOnDelay NoInit9/1 -> Associated TCMS Fault ID41/1(State)
  TimerOnDelay NoInit10/1 -> Associated TCMS Fault ID45/1(State)
  TimerOnDelay NoInit11/1 -> Associated TCMS Fault ID43/1(State)
  TimerOnDelay NoInit12/1 -> Associated TCMS Fault ID44/1(State)
  TimerOnDelay NoInit13/1 -> Associated TCMS Fault ID48/1(State)
  TimerOnDelay NoInit14/1 -> Associated TCMS Fault ID46/1(State)
  TimerOnDelay NoInit15/1 -> Associated TCMS Fault ID47/1(State)
  TimerOnDelay NoInit16/1 -> Associated TCMS Fault ID51/1(State)
  TimerOnDelay NoInit17/1 -> Associated TCMS Fault ID49/1(State)
  TimerOnDelay NoInit18/1 -> Associated TCMS Fault ID50/1(State)
  TimerOnDelay NoInit19/1 -> Associated TCMS Fault ID54/1(State)
  TimerOnDelay NoInit20/1 -> Associated TCMS Fault ID52/1(State)
  TimerOnDelay NoInit21/1 -> Associated TCMS Fault ID53/1(State)
  TimerOnDelay NoInit22/1 -> Associated TCMS Fault ID57/1(State)
  TimerOnDelay NoInit23/1 -> Associated TCMS Fault ID1/1(State)

== system TCMSSystem/TCMSSystemPerVehicle/EnabledTCMSVehicle/TCMSDoors/DoorsDisplay/CabTrainDisplay/CabActiveTrainDisplay ==
  In Bus Element : Inport  PortName=ElectricalSignals  Element=AllLeftDoorsClosed
  In Bus Element1 : Inport  PortName=ElectricalSignals  Element=AllRightDoorsClosed
  Action Port : ActionPort  ActionPortLabel=if(u1 > 0)
  AND : Logic  AllPortsSameDT=off  OutDataTypeStr=boolean
  Bus Creator : BusCreator  Inputs=3
  Data Type Conversion : DataTypeConversion  OutDataTypeStr=double
  Data Type Conversion1 : DataTypeConversion  OutDataTypeStr=double
  Data Type Conversion2 : DataTypeConversion  OutDataTypeStr=double
  Out1 : Outport
  wires:
  Data Type Conversion2/1 -> Bus Creator/3  "AllDoorsClosed"
  Data Type Conversion1/1 -> Bus Creator/2  "AllLeftDoorsClosed"
  Data Type Conversion/1 -> Bus Creator/1  "AllRightDoorsClosed"
  In Bus Element/1 -> AND/2, Data Type Conversion1/1
  In Bus Element1/1 -> AND/1, Data Type Conversion/1
  Bus Creator/1 -> Out1/1
  AND/1 -> Data Type Conversion2/1

== system TCMSSystem/TCMSSystemPerVehicle/EnabledTCMSVehicle/TCMSDoors/DoorsDisplay/CabTrainDisplay/CabInactiveNoDisplay ==
  Action Port : ActionPort  ActionPortLabel=else
  Bus Creator : BusCreator  Inputs=3
  Constant : Constant  Value=0
  Constant1 : Constant  Value=0
  Constant2 : Constant  Value=0
  Out1 : Outport
  wires:
  Constant2/1 -> Bus Creator/3  "AllDoorsClosed"
  Constant1/1 -> Bus Creator/2  "AllLeftDoorsClosed"
  Constant/1 -> Bus Creator/1  "AllRightDoorsClosed"
  Bus Creator/1 -> Out1/1

== system TCMSSystem/TCMSSystemPerVehicle/EnabledTCMSVehicle/TCMSDoors/DoorsDisplay/TCMSVehicleInfo/DoorsStatus1 ==
  Doors : Inport  Partition=on  PartitionDimension=1  PartitionWidth=1  PartitionOffset=0
  Bus Selector : BusSelector  OutputSignals=DoorClosedStatus,DoorOpenStatus,DoorReleasedAuthorisedToOpenStatus,DoorEmergencyReleasedStatus,DoorIsolatedStatus,DoorFaultStatus,DoorObstacleDetected,DoorObstacleUnableToClose,DoorLockedStatus,DoorCloseObstruction,DoorOpenObstruction,DoorMotorCircuitFailure,DoorFailedToLock,DoorFailedToUnlock,DoorUnexpectedUnlocking,DCUFailure,DCSRFailure,DCSLFailure,DLSRFailure,DLSLFailure,DoorMajorFault,UnexpectedDoorOpeningDetectedByCC
  Data Type Conversion{,1..8} (9 alike) : DataTypeConversion  OutDataTypeStr=double
  For Each : ForEach  DisableCoverage=on
  Terminator{,1..3} (4 alike) : Terminator
  DoorOpenStatus : Outport  ConcatenationDimension=1
  DoorEmergencyReleasedStatus : Outport  Port=2  ConcatenationDimension=1
  DoorIsolatedStatus : Outport  Port=3  ConcatenationDimension=1
  DoorFaultStatus : Outport  Port=4  ConcatenationDimension=1
  DoorLockedStatus : Outport  Port=5  ConcatenationDimension=1
  DoorCloseObstruction : Outport  Port=6  ConcatenationDimension=1
  DoorOpenObstruction : Outport  Port=7  ConcatenationDimension=1
  DoorMotorCircuitFailure : Outport  Port=8  ConcatenationDimension=1
  DoorFailedToLock : Outport  Port=9  ConcatenationDimension=1
  DoorFailedToUnlock : Outport  Port=10  ConcatenationDimension=1
  DoorUnexpectedUnlocking : Outport  Port=11  ConcatenationDimension=1
  DCUFailure : Outport  Port=12  ConcatenationDimension=1
  DCSRFailure : Outport  Port=13  ConcatenationDimension=1
  DCSLFailure : Outport  Port=14  ConcatenationDimension=1
  DLSRFailure : Outport  Port=15  ConcatenationDimension=1
  DLSLFailure : Outport  Port=16  ConcatenationDimension=1
  DoorMajorFault : Outport  Port=17  ConcatenationDimension=1
  UnexpectedDoorOpeningDetectedByCC : Outport  Port=18  ConcatenationDimension=1
  wires:
  Bus Selector/8 -> Data Type Conversion5/1  "<DoorObstacleUnableToClose>"
  Bus Selector/2 -> Data Type Conversion3/1  "<DoorOpenStatus>"
  Bus Selector/1 -> Data Type Conversion4/1  "<DoorClosedStatus>"
  Bus Selector/4 -> Data Type Conversion1/1  "<DoorEmergencyReleasedStatus>"
  Bus Selector/6 -> Data Type Conversion7/1  "<DoorFaultStatus>"
  Bus Selector/7 -> Data Type Conversion6/1  "<DoorObstacleDetected>"
  Bus Selector/5 -> Data Type Conversion/1  "<DoorIsolatedStatus>"
  Bus Selector/3 -> Data Type Conversion2/1  "<DoorReleasedAuthorisedToOpenStatus>"
  Doors/1 -> Bus Selector/1
  Bus Selector/9 -> Data Type Conversion8/1  "<DoorLockedStatus>"
  Data Type Conversion4/1 -> Terminator/1  "DoorClosedStatus"
  Data Type Conversion2/1 -> Terminator1/1  "DoorReleasedAuthorisedToOpenStatus"
  Data Type Conversion6/1 -> Terminator2/1  "DoorObstacleDetected"
  Data Type Conversion5/1 -> Terminator3/1  "DoorObstacleUnableToClose"
  Data Type Conversion3/1 -> DoorOpenStatus/1  "DoorOpenStatus"
  Data Type Conversion1/1 -> DoorEmergencyReleasedStatus/1  "DoorEmergencyReleasedStatus"
  Data Type Conversion8/1 -> DoorLockedStatus/1  "DoorLockedStatus"
  Data Type Conversion/1 -> DoorIsolatedStatus/1  "DoorIsolatedStatus"
  Data Type Conversion7/1 -> DoorFaultStatus/1  "DoorFaultStatus"
  Bus Selector/11 -> DoorOpenObstruction/1  "<DoorOpenObstruction>"
  Bus Selector/10 -> DoorCloseObstruction/1  "<DoorCloseObstruction>"
  Bus Selector/12 -> DoorMotorCircuitFailure/1  "<DoorMotorCircuitFailure>"
  Bus Selector/13 -> DoorFailedToLock/1  "<DoorFailedToLock>"
  Bus Selector/14 -> DoorFailedToUnlock/1  "<DoorFailedToUnlock>"
  Bus Selector/15 -> DoorUnexpectedUnlocking/1  "<DoorUnexpectedUnlocking>"
  Bus Selector/16 -> DCUFailure/1  "<DCUFailure>"
  Bus Selector/17 -> DCSRFailure/1  "<DCSRFailure>"
  Bus Selector/18 -> DCSLFailure/1  "<DCSLFailure>"
  Bus Selector/19 -> DLSRFailure/1  "<DLSRFailure>"
  Bus Selector/20 -> DLSLFailure/1  "<DLSLFailure>"
  Bus Selector/21 -> DoorMajorFault/1  "<DoorMajorFault>"
  Bus Selector/22 -> UnexpectedDoorOpeningDetectedByCC/1  "<UnexpectedDoorOpeningDetectedByCC>"
